simulink model "Digital_CityBus"  (R2020a)
settings: Solver=FixedStepDiscrete  StartTime=0.0  StopTime=10  FixedStep=1  RelTol=1e-3
model workspace (MAT data in the model file):
  Destination_Code = Simulink.Signal
  Destination_Code.Description = 'Entered Destination code for ticket generation'
  Destination_Code.DataType = 'single'
  Destination_Code.Min = 1
  Destination_Code.Max = 4
  Destination_Code.Dimensions = -1
  Destination_Code.DimensionsMode = 'auto'
  Destination_Code.Complexity = 'auto'
  Destination_Code.SampleTime = -1
  Destination_Code.SamplingMode = 'auto'
  Destination_St_Codes = Simulink.Parameter
  Destination_St_Codes.Value = [0 1 2 3 4]
  Destination_St_Codes.Description = 'For Each Station there is code Which is helpful while 
    | Generating Tickets for Passengers.
    | Bus is traveling from Swargate To Katraj in Pune
    | So Code for stations are
    | 
    | 0 for Swargate
    | 1 for City_Pride
    | 2 for Balaji_Nagar
    | 3 for Bharthi_Vidhyapith
    | 4 for Katraj
    | 
    | from one station to next station need 5rs for one Passenger 
    | for example one passenger want go from swargate to katraj
    | he need 25rs'
  Destination_St_Codes.DataType = 'uint8'
  Destination_St_Codes.Min = 0
  Destination_St_Codes.Max = 4
  Destination_St_Codes.Dimensions = [1 5]
  Entering_Passengers = Simulink.Signal
  Entering_Passengers.Description = 'Number Of Passengers Entering into Bus at Boarding Station of Passengers 
    | And Limitation is One Passenger At Time Also Maximum Passenger Enter into
    | Bus is 50 One By One'
  Entering_Passengers.DataType = 'uint8'
  Entering_Passengers.Min = 0
  Entering_Passengers.Max = 50
  Entering_Passengers.Dimensions = -1
  Entering_Passengers.DimensionsMode = 'auto'
  Entering_Passengers.Complexity = 'auto'
  Entering_Passengers.SampleTime = -1
  Entering_Passengers.SamplingMode = 'auto'
  Leaving_Passengers = Simulink.Signal
  Leaving_Passengers.Description = 'Number of Passengers Leaving The Bus At Destination Station of That 
    | Passengers From Back Door of The Bus But Passengers Should Leave the One
    | by one not all at time'
  Leaving_Passengers.DataType = 'uint8'
  Leaving_Passengers.Min = 0
  Leaving_Passengers.Max = 50
  Leaving_Passengers.Dimensions = -1
  Leaving_Passengers.DimensionsMode = 'auto'
  Leaving_Passengers.Complexity = 'auto'
  Leaving_Passengers.SampleTime = -1
  Leaving_Passengers.SamplingMode = 'auto'
  Max_Seats = Simulink.Parameter
  Max_Seats.Value = 50
  Max_Seats.Description = 'Maximum Passengers can  Enters in Bus is 50 only'
  Max_Seats.DataType = 'uint8'
  Max_Seats.Min = 0
  Max_Seats.Max = 50
  Max_Seats.Dimensions = [1 1]
  Number_Of_Passengers = Simulink.Signal
  Number_Of_Passengers.Description = 'Number of passengers are entered in Perticular station
    | for them need to generate Tickets.
    | from one station to next station need 10rs
    | '
  Number_Of_Passengers.DataType = 'uint8'
  Number_Of_Passengers.Min = 1
  Number_Of_Passengers.Max = 50
  Number_Of_Passengers.Dimensions = -1
  Number_Of_Passengers.DimensionsMode = 'auto'
  Number_Of_Passengers.Complexity = 'auto'
  Number_Of_Passengers.SampleTime = -1
  Number_Of_Passengers.SamplingMode = 'auto'
  Present_Passengers = Simulink.Signal
  Present_Passengers.Description = 'Present Passengers in Bus'
  Present_Passengers.DataType = 'uint8'
  Present_Passengers.Min = 0
  Present_Passengers.Max = 50
  Present_Passengers.Dimensions = -1
  Present_Passengers.DimensionsMode = 'auto'
  Present_Passengers.Complexity = 'real'
  Present_Passengers.SampleTime = -1
  Present_Passengers.SamplingMode = 'auto'
  TOTAL_SEATS = 50
  Tickets_Price = Simulink.Parameter
  Tickets_Price.Value = [0 5 10 15 20]
  Tickets_Price.Description = 'Bus is traveling from Swargate To Katraj in Pune
    | So Code for stations are
    | 
    | 0 for Swargate
    | 1 for City_Pride
    | 2 for Balaji_Nagar
    | 3 for Bharthi_Vidhyapith
    | 4 for Katraj
    | 
    | from one station to next station need 5rs for one Passenger 
    | for example one passenger want go from swargate to katraj
    | he need 25rs'
  Tickets_Price.DataType = 'uint8'
  Tickets_Price.DocUnits = 'Rupee'
  Tickets_Price.Dimensions = [1 5]
undefined symbols (not defined in the file): Back_Door_Status, Bus_Traveling_Route, Generated_Ticket, Seats_Status, Total_Cash_Collection
libraries: simulink x4
settings Model: OrderedModelArguments=off  Creator=sagar  LastModifiedBy=Ganesh
settings SolverCC: AlgebraicLoopSolver=LineSearch
settings DataIOCC: ReturnWorkspaceOutputs=off
settings DebuggingCC: ArithmeticOperatorsInVariantConditions=warning
settings SFSimCC: SimUseLocalCustomCode=off  CustomCodeUndefinedFunction=UseInterfaceOnly
settings RTWCC: RTWUseLocalCustomCode=off

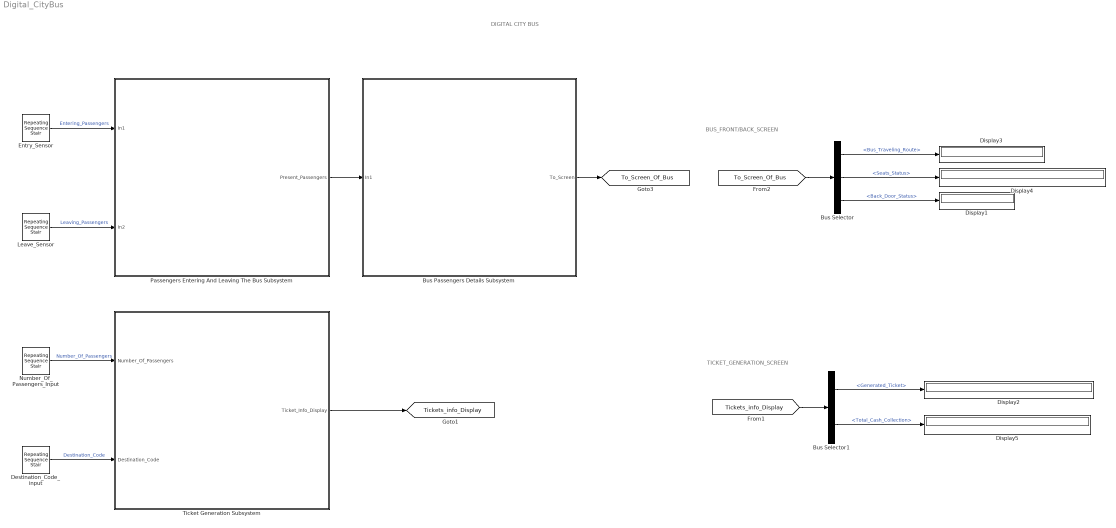
== system Digital_CityBus ==
  note: DIGITAL CITY BUS
  note: TICKET_GENERATION_SCREEN
  note: BUS_FRONT/BACK_SCREEN
  Bus Selector : BusSelector  OutputSignals=Bus_Traveling_Route,Seats_Status,Back_Door_Status
  Bus Selector1 : BusSelector  OutputSignals=Generated_Ticket,Total_Cash_Collection
  Bus Passengers Details Subsystem : Subsystem
      mask Display: image('$imagefile'); % Use "Edit Image" on toolstrip to change.
  Destination_Code_input : simulink/Sources/Repeating Sequence Stair  OutValues=[4].'  tsamp=-1  OutMin=[0]  OutMax=[50]  OutDataTypeStr=single  OutputDataTypeScalingMode=single  OutDataType=fixdt(0,8)  ConRadixGroup=Best Precision: Vector-wise  OutScaling=2^-12
  Display{1..5} (5 alike) : Display
  Entry_Sensor : simulink/Sources/Repeating Sequence Stair  OutValues=[1]  tsamp=-1  OutMin=[0]  OutMax=[50]  OutDataTypeStr=uint8  OutputDataTypeScalingMode=uint8  OutDataType=fixdt(0,8)  ConRadixGroup=Best Precision: Vector-wise  OutScaling=2^-12
  Leave_Sensor : simulink/Sources/Repeating Sequence Stair  OutValues=[0].'  tsamp=-1  OutMin=[0]  OutMax=[50]  OutDataTypeStr=uint8  OutputDataTypeScalingMode=uint8  OutDataType=fixdt(0,8)  ConRadixGroup=Best Precision: Vector-wise  OutScaling=2^-12
  Number_Of_Passengers_Input : simulink/Sources/Repeating Sequence Stair  OutValues=[1]  tsamp=-1  OutMin=[0]  OutMax=[50]  OutDataTypeStr=uint8  OutputDataTypeScalingMode=uint8  OutDataType=fixdt(0,8)  ConRadixGroup=Best Precision: Vector-wise  OutScaling=2^-12
  Passengers Entering And Leaving The Bus Subsystem : Subsystem  TreatAsAtomicUnit=on
      mask Display: image('bus.png'); % Use "Edit Image" on toolstrip to change.
  Ticket Generation Subsystem : Subsystem
      mask Display: image('tickets.png'); % Use "Edit Image" on toolstrip to change.
  tag scope: Tickets_info_Display=global, To_Screen_Of_Bus=global
  wires:
  Bus Selector/3 -> Display1/1  "<Back_Door_Status>"
  Bus Selector/2 -> Display4/1  "<Seats_Status>"
  Bus Selector/1 -> Display3/1  "<Bus_Traveling_Route>"
  [To_Screen_Of_Bus] -> Bus Selector/1
  Bus Passengers Details Subsystem/1(To_Screen) -> [To_Screen_Of_Bus]
  Entry_Sensor/1 -> Passengers Entering And Leaving The Bus Subsystem/1(In1)  "Entering_Passengers"
  Leave_Sensor/1 -> Passengers Entering And Leaving The Bus Subsystem/2(In2)  "Leaving_Passengers"
  Number_Of_Passengers_Input/1 -> Ticket Generation Subsystem/1(Number_Of_Passengers)  "Number_Of_Passengers"
  Destination_Code_input/1 -> Ticket Generation Subsystem/2(Destination_Code)  "Destination_Code"
  Bus Selector1/1 -> Display2/1  "<Generated_Ticket>"
  Bus Selector1/2 -> Display5/1  "<Total_Cash_Collection>"
  Ticket Generation Subsystem/1(Ticket_Info_Display) -> [Tickets_info_Display]
  [Tickets_info_Display] -> Bus Selector1/1
  Passengers Entering And Leaving The Bus Subsystem/1(Present_Passengers) -> Bus Passengers Details Subsystem/1(In1)

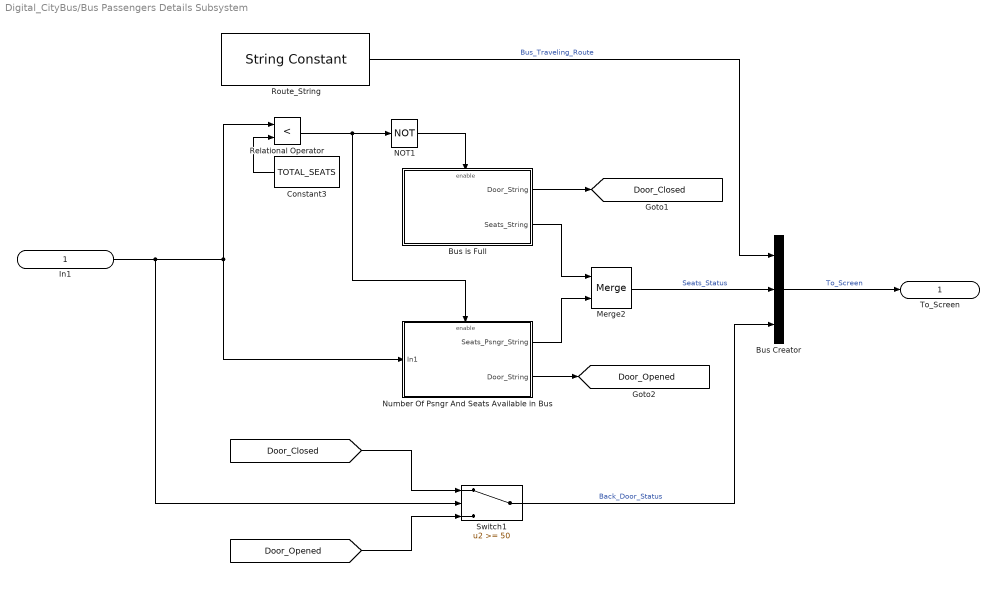
== system Digital_CityBus/Bus Passengers Details Subsystem ==
  In1 : Inport
  Bus Creator : BusCreator  Inputs=Bus_Traveling_Route,Seats_Status,Back_Door_Status
  Bus is Full : Subsystem  TreatAsAtomicUnit=on
  Constant3 : Constant  Value=TOTAL_SEATS
  Merge2 : Merge
  NOT1 : Logic  Operator=NOT  IconShape=distinctive  AllPortsSameDT=off  OutDataTypeStr=boolean
  Number Of Psngr And Seats Available in Bus : Subsystem  TreatAsAtomicUnit=on
  Relational Operator : RelationalOperator  Operator=<  OutDataTypeStr=boolean  RndMeth=Simplest
  Route_String : StringConstant  String="\"Bus From Swargate To Katraj\""
  Switch1 : Switch  Threshold=50
      settings: AttributesFormatString=MAX_SEATS=%<Threshold>
  To_Screen : Outport  VectorParamsAs1DForOutWhenUnconnected=off
  tag scope: Door_Closed=global, Door_Opened=global
  wires:
  Constant3/1 -> Relational Operator/2
  Bus is Full/2(Seats_String) -> Merge2/1
  In1/1 -> Switch1/2, Relational Operator/1, Number Of Psngr And Seats Available in Bus/1(In1)
  NOT1/1 -> Bus is Full/Enable
  Bus is Full/1(Door_String) -> [Door_Closed]
  Number Of Psngr And Seats Available in Bus/1(Seats_Psngr_String) -> Merge2/2
  Merge2/1 -> Bus Creator/2  "Seats_Status"
  Switch1/1 -> Bus Creator/3  "Back_Door_Status"
  Number Of Psngr And Seats Available in Bus/2(Door_String) -> [Door_Opened]
  Relational Operator/1 -> Number Of Psngr And Seats Available in Bus/Enable, NOT1/1
  Route_String/1 -> Bus Creator/1  "Bus_Traveling_Route"
  [Door_Closed] -> Switch1/1
  [Door_Opened] -> Switch1/3
  Bus Creator/1 -> To_Screen/1  "To_Screen"

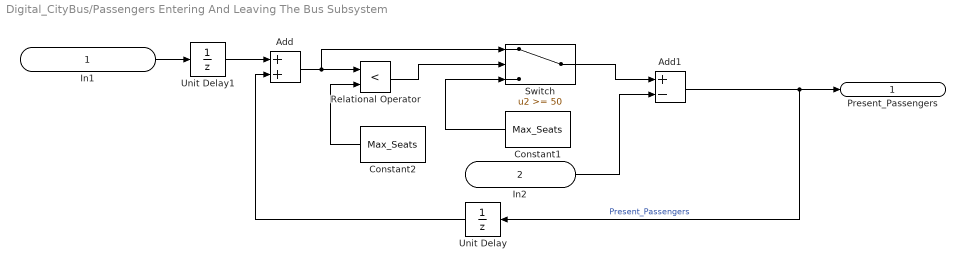
== system Digital_CityBus/Passengers Entering And Leaving The Bus Subsystem ==
  In1 : Inport
  In2 : Inport  Port=2
  Add : Sum
  Add1 : Sum  Inputs=+-
  Constant1 : Constant  Value=Max_Seats
  Constant2 : Constant  Value=Max_Seats
  Relational Operator : RelationalOperator  Operator=<  OutDataTypeStr=boolean  RndMeth=Simplest
  Switch : Switch  Threshold=50
  Unit Delay : UnitDelay  SampleTime=-1  HasFrameUpgradeWarning=on
  Unit Delay1 : UnitDelay  SampleTime=-1  HasFrameUpgradeWarning=on
  Present_Passengers : Outport  VectorParamsAs1DForOutWhenUnconnected=off
  wires:
  Add1/1 -> Present_Passengers/1, Unit Delay/1  "Present_Passengers"
  Unit Delay/1 -> Add/2
  Add/1 -> Relational Operator/1, Switch/1
  In2/1 -> Add1/2
  Switch/1 -> Add1/1
  In1/1 -> Unit Delay1/1
  Constant2/1 -> Relational Operator/2
  Relational Operator/1 -> Switch/2
  Constant1/1 -> Switch/3
  Unit Delay1/1 -> Add/1

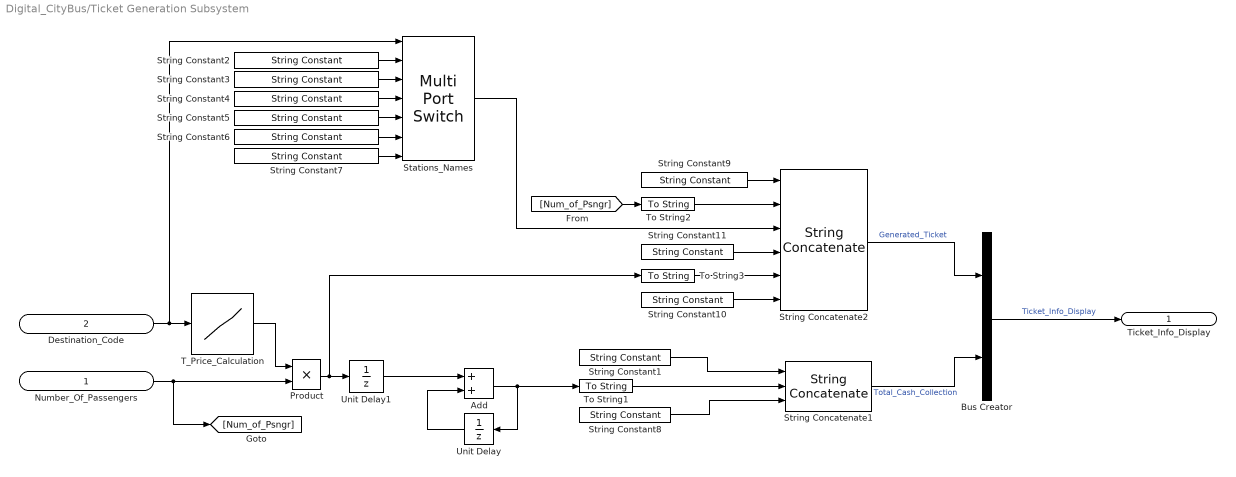
== system Digital_CityBus/Ticket Generation Subsystem ==
  Number_Of_Passengers : Inport
  Destination_Code : Inport  Port=2
  Add : Sum
  Bus Creator : BusCreator  Inputs=Generated_Ticket,Total_Cash_Collection
  Product : Product
  Stations_Names : MultiPortSwitch  DataPortOrder=Zero-based contiguous  Inputs=6  DiagnosticForDefault=None  zeroidx=on
  String Concatenate1 : StringConcatenate  Inputs=3
  String Concatenate2 : StringConcatenate  Inputs=6
  String Constant1 : StringConstant  String="\" Total Collection is=\""
  String Constant10 : StringConstant  String="\"Rs\""
  String Constant11 : StringConstant  String="\"  amount=\""
  String Constant2 : StringConstant  String="\"  Destination Swargate  \""
  String Constant3 : StringConstant  String="\"  Destination City Pride  \""
  String Constant4 : StringConstant  String="\"  Destination Balaji Nagar  \""
  String Constant5 : StringConstant  String="\"  Destination Bharti Vidhyapith  \""
  String Constant6 : StringConstant  String="\"  Destination Katraj  \""
  String Constant7 : StringConstant  String="\"  Invalied Station  \""
  String Constant8 : StringConstant  String="\" Rs\""
  String Constant9 : StringConstant  String="\"No. Of Passengers is \""
  T_Price_Calculation : Lookup_n-D  NumberOfTableDimensions=1  BreakpointsForDimension1=Destination_St_Codes  Table=Tickets_Price  InternalRulePriority=Speed  RndMeth=Simplest  InputSameDT=on
  To String1 : ToString
  To String2 : ToString
  To String3 : ToString
  Unit Delay : UnitDelay  SampleTime=-1  HasFrameUpgradeWarning=on
  Unit Delay1 : UnitDelay  SampleTime=-1  HasFrameUpgradeWarning=on
  Ticket_Info_Display : Outport  VectorParamsAs1DForOutWhenUnconnected=off
  wires:
  Destination_Code/1 -> Stations_Names/1, T_Price_Calculation/1
  Unit Delay/1 -> Add/2
  Add/1 -> Unit Delay/1, To String1/1
  Unit Delay1/1 -> Add/1
  Product/1 -> To String3/1, Unit Delay1/1
  String Constant1/1 -> String Concatenate1/1
  String Constant2/1 -> Stations_Names/2
  String Constant3/1 -> Stations_Names/3
  String Constant4/1 -> Stations_Names/4
  String Constant5/1 -> Stations_Names/5
  String Constant6/1 -> Stations_Names/6
  T_Price_Calculation/1 -> Product/1
  Number_Of_Passengers/1 -> Product/2, [Num_of_Psngr]
  String Constant7/1 -> Stations_Names/7
  To String1/1 -> String Concatenate1/2
  String Constant8/1 -> String Concatenate1/3
  [Num_of_Psngr] -> To String2/1
  String Concatenate2/1 -> Bus Creator/1  "Generated_Ticket"
  String Concatenate1/1 -> Bus Creator/2  "Total_Cash_Collection"
  Bus Creator/1 -> Ticket_Info_Display/1  "Ticket_Info_Display"
  String Constant10/1 -> String Concatenate2/6
  To String3/1 -> String Concatenate2/5
  String Constant11/1 -> String Concatenate2/4
  String Constant9/1 -> String Concatenate2/1
  To String2/1 -> String Concatenate2/2
  Stations_Names/1 -> String Concatenate2/3

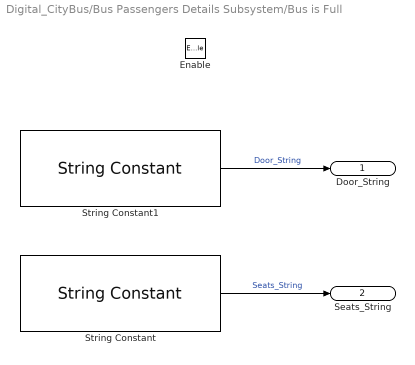
== system Digital_CityBus/Bus Passengers Details Subsystem/Bus is Full ==
  "Enable " : EnablePort  StatesWhenEnabling=reset
  String Constant : StringConstant  String="\"All Seats are Full\""
  String Constant1 : StringConstant  String="\"Back Door is Closed\""
  Door_String : Outport  VectorParamsAs1DForOutWhenUnconnected=off
  Seats_String : Outport  Port=2  VectorParamsAs1DForOutWhenUnconnected=off
  wires:
  String Constant/1 -> Seats_String/1  "Seats_String"
  String Constant1/1 -> Door_String/1  "Door_String"

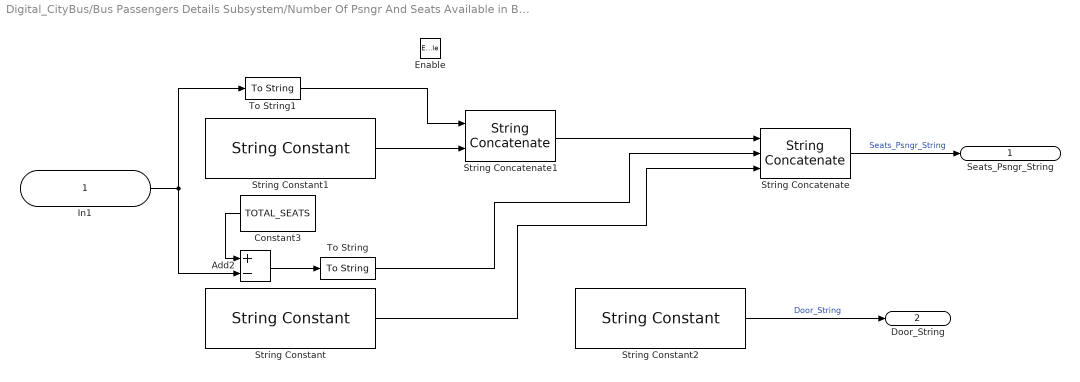
== system Digital_CityBus/Bus Passengers Details Subsystem/Number Of Psngr And Seats Available in Bus ==
  In1 : Inport
  Enable : EnablePort
  Add2 : Sum  Inputs=+-
  Constant3 : Constant  Value=TOTAL_SEATS
  String Concatenate : StringConcatenate  Inputs=3
  String Concatenate1 : StringConcatenate
  String Constant : StringConstant  String="\" Seats are available\""
  String Constant1 : StringConstant  String="\" Passengers Present in Bus And \""
  String Constant2 : StringConstant  String="\"Back Door is Opened\""
  To String : ToString
  To String1 : ToString
  Seats_Psngr_String : Outport  VectorParamsAs1DForOutWhenUnconnected=off
  Door_String : Outport  Port=2  VectorParamsAs1DForOutWhenUnconnected=off
  wires:
  Add2/1 -> To String/1
  In1/1 -> Add2/2, To String1/1
  String Constant/1 -> String Concatenate/3
  To String/1 -> String Concatenate/2
  String Constant1/1 -> String Concatenate1/2
  String Concatenate1/1 -> String Concatenate/1
  To String1/1 -> String Concatenate1/1
  Constant3/1 -> Add2/1
  String Constant2/1 -> Door_String/1  "Door_String"
  String Concatenate/1 -> Seats_Psngr_String/1  "Seats_Psngr_String"
